simulink model "fig434sim"  (Simulink 3.00)
settings: Solver=ode45  SolverMode=SingleTasking  StartTime=0.0  StopTime=5  RelTol=1e-3  AbsTol=1e-6
undefined symbols (not defined in the file or in its folder): denD, numD, T
libraries: simulink3 x2

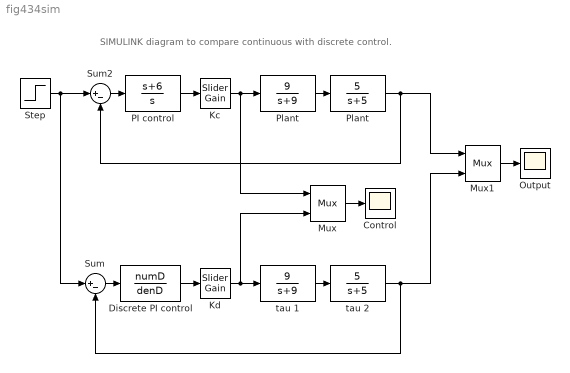
== system fig434sim ==
  note: SIMULINK diagram to compare continuous with discrete control.
  Control : Scope
      settings: TickLabels=on  TimeRange=auto  YMin=0  YMax=2.75  SaveName=ucd  DataFormat=Matrix
  Discrete PI control : DiscreteTransferFcn  Numerator=numD  Denominator=denD  SampleTime=T
  Kc : simulink3/Math/Slider Gain  low=0  gain=1.4  high=10
  Kd : simulink3/Math/Slider Gain  low=0  gain=1.4  high=10
  Mux : Mux  Inputs=2
      settings: DisplayOption=none
  Mux1 : Mux  Inputs=2
      settings: DisplayOption=none
  Output : Scope
      settings: TickLabels=on  TimeRange=auto  YMin=-5  YMax=5  SaveName=ycd  DataFormat=Matrix
  PI control : TransferFcn  Numerator=[1 6]  Denominator=[1 0]
  Plant : TransferFcn  Numerator=[9]  Denominator=[1 9]
  "Plant " : TransferFcn  Numerator=[5]  Denominator=[1 5]
  Step : Step  Time=.1  Before=0  After=1  SampleTime=.001
  Sum : Sum  Inputs=|+-  SaturateOnIntegerOverflow=off
  Sum2 : Sum  Inputs=|+-  SaturateOnIntegerOverflow=off
  tau 1 : TransferFcn  Numerator=[9]  Denominator=[1 9]
  tau 2 : TransferFcn  Numerator=[5]  Denominator=[1 5]
  wires:
  PI control/1 -> Kc/1
  Sum2/1 -> PI control/1
  Plant/1 -> "Plant "/1
  Discrete PI control/1 -> Kd/1
  tau 1/1 -> tau 2/1
  Step/1 -> Sum2/1, Sum/1
  Kc/1 -> Plant/1, Mux/1
  Mux/1 -> Control/1
  "Plant "/1 -> Mux1/1, Sum2/2
  Mux1/1 -> Output/1
  Sum/1 -> Discrete PI control/1
  Kd/1 -> tau 1/1, Mux/2
  tau 2/1 -> Mux1/2, Sum/2
